simulink model "AUV_MechanicsFullHydrodynamicsVAR"  (R2020b)
settings: Solver=ode23t  StartTime=0.0  StopTime=60  MaxStep=0.01  RelTol=1e-3  EnableMultiTasking=on
PreLoadFcn:
  | AUV_VehicleParameters;
  | Vehicle.Body.markeropacity = 0;
StartFcn:
  | tic;
StopFcn:
  | toc;
model workspace: external: MATLAB File AUV_DataFile_ORIG.m (data not in the file)
undefined symbols (not defined in the file): Environment, Newton, Raphson, smiData, x, X, Y, y, Z
libraries: sm_lib x1595, nesl_utility x51, sharedutil x8, AUVCustomPrimitives_Lib x4, shared6dof x1, aerolibasang x1, aerolibadyn x1
(part 2 of 33)

== system AUV_MechanicsFullHydrodynamicsVAR/AUV/Muiltibody/Cameras ==
  Behind : sm_lib/Frames and Transforms/Reference Frame
  BehindDown : sm_lib/Frames and Transforms/Reference Frame
  BehindUP : sm_lib/Frames and Transforms/Reference Frame
  BehindUPLeft : sm_lib/Frames and Transforms/Reference Frame
  BehindUPRight : sm_lib/Frames and Transforms/Reference Frame
  Side : sm_lib/Frames and Transforms/Reference Frame
  T1 : sm_lib/Frames and Transforms/Rigid Transform  TranslationMethod=Cartesian  TranslationStandardOffset=0  TranslationLengthUnit=m  TranslationStandardAxis=+Z  TranslationCartesianOffset=[-3 0 0]  TranslationROffset=0  TranslationROffsetUnits=m  TranslationZOffset=0  TranslationZOffsetUnits=m  TranslationThetaOffset=0  TranslationThetaOffsetUnits=deg  RotationMethod=None  RotationAngleUnits=deg  RotationStandardAxis=+Z  RotationAngle=0.0  RotationArbitraryAxis=[0 0 1]  FollAlignAxisA=+X  BaseAlignAxisA=+Y  FollAlignAxisB=+Y  BaseAlignAxisB=+Z  RotationSequenceAxes=FollowerAxes  RotationSequence=XYX  RotationSequenceAngles=[0 0 0]  RotationSequenceAnglesUnits=deg  RotationMatrix=[1 0 0; 0 1 0; 0 0 1]
  T2 : sm_lib/Frames and Transforms/Rigid Transform  TranslationMethod=Cartesian  TranslationStandardOffset=0  TranslationLengthUnit=m  TranslationStandardAxis=+Z  TranslationCartesianOffset=[0 0 -3]  TranslationROffset=0  TranslationROffsetUnits=m  TranslationZOffset=0  TranslationZOffsetUnits=m  TranslationThetaOffset=0  TranslationThetaOffsetUnits=deg  RotationMethod=None  RotationAngleUnits=deg  RotationStandardAxis=+Z  RotationAngle=0.0  RotationArbitraryAxis=[0 0 1]  FollAlignAxisA=+X  BaseAlignAxisA=+Y  FollAlignAxisB=+Y  BaseAlignAxisB=+Z  RotationSequenceAxes=FollowerAxes  RotationSequence=XYX  RotationSequenceAngles=[0 0 0]  RotationSequenceAnglesUnits=deg  RotationMatrix=[1 0 0; 0 1 0; 0 0 1]
  T3 : sm_lib/Frames and Transforms/Rigid Transform  TranslationMethod=Cartesian  TranslationStandardOffset=0  TranslationLengthUnit=m  TranslationStandardAxis=+Z  TranslationCartesianOffset=[0 0 -3]  TranslationROffset=0  TranslationROffsetUnits=m  TranslationZOffset=0  TranslationZOffsetUnits=m  TranslationThetaOffset=0  TranslationThetaOffsetUnits=deg  RotationMethod=None  RotationAngleUnits=deg  RotationStandardAxis=+Z  RotationAngle=0.0  RotationArbitraryAxis=[0 0 1]  FollAlignAxisA=+X  BaseAlignAxisA=+Y  FollAlignAxisB=+Y  BaseAlignAxisB=+Z  RotationSequenceAxes=FollowerAxes  RotationSequence=XYX  RotationSequenceAngles=[0 0 0]  RotationSequenceAnglesUnits=deg  RotationMatrix=[1 0 0; 0 1 0; 0 0 1]
  T4 : sm_lib/Frames and Transforms/Rigid Transform  TranslationMethod=Cartesian  TranslationStandardOffset=0  TranslationLengthUnit=m  TranslationStandardAxis=+Z  TranslationCartesianOffset=[0 -2 0]  TranslationROffset=0  TranslationROffsetUnits=m  TranslationZOffset=0  TranslationZOffsetUnits=m  TranslationThetaOffset=0  TranslationThetaOffsetUnits=deg  RotationMethod=None  RotationAngleUnits=deg  RotationStandardAxis=+Z  RotationAngle=0.0  RotationArbitraryAxis=[0 0 1]  FollAlignAxisA=+X  BaseAlignAxisA=+Y  FollAlignAxisB=+Y  BaseAlignAxisB=+Z  RotationSequenceAxes=FollowerAxes  RotationSequence=XYX  RotationSequenceAngles=[0 0 0]  RotationSequenceAnglesUnits=deg  RotationMatrix=[1 0 0; 0 1 0; 0 0 1]
  T5 : sm_lib/Frames and Transforms/Rigid Transform  TranslationMethod=Cartesian  TranslationStandardOffset=0  TranslationLengthUnit=m  TranslationStandardAxis=+Z  TranslationCartesianOffset=[0 -2 0]  TranslationROffset=0  TranslationROffsetUnits=m  TranslationZOffset=0  TranslationZOffsetUnits=m  TranslationThetaOffset=0  TranslationThetaOffsetUnits=deg  RotationMethod=None  RotationAngleUnits=deg  RotationStandardAxis=+Z  RotationAngle=0.0  RotationArbitraryAxis=[0 0 1]  FollAlignAxisA=+X  BaseAlignAxisA=+Y  FollAlignAxisB=+Y  BaseAlignAxisB=+Z  RotationSequenceAxes=FollowerAxes  RotationSequence=XYX  RotationSequenceAngles=[0 0 0]  RotationSequenceAnglesUnits=deg  RotationMatrix=[1 0 0; 0 1 0; 0 0 1]
  T6 : sm_lib/Frames and Transforms/Rigid Transform  TranslationMethod=Cartesian  TranslationStandardOffset=0  TranslationLengthUnit=m  TranslationStandardAxis=+Z  TranslationCartesianOffset=[0 0 -3]  TranslationROffset=0  TranslationROffsetUnits=m  TranslationZOffset=0  TranslationZOffsetUnits=m  TranslationThetaOffset=0  TranslationThetaOffsetUnits=deg  RotationMethod=None  RotationAngleUnits=deg  RotationStandardAxis=+Z  RotationAngle=0.0  RotationArbitraryAxis=[0 0 1]  FollAlignAxisA=+X  BaseAlignAxisA=+Y  FollAlignAxisB=+Y  BaseAlignAxisB=+Z  RotationSequenceAxes=FollowerAxes  RotationSequence=XYX  RotationSequenceAngles=[0 0 0]  RotationSequenceAnglesUnits=deg  RotationMatrix=[1 0 0; 0 1 0; 0 0 1]
  T7 : sm_lib/Frames and Transforms/Rigid Transform  TranslationMethod=Cartesian  TranslationStandardOffset=0  TranslationLengthUnit=m  TranslationStandardAxis=+Z  TranslationCartesianOffset=[0 -3 0]  TranslationROffset=0  TranslationROffsetUnits=m  TranslationZOffset=0  TranslationZOffsetUnits=m  TranslationThetaOffset=0  TranslationThetaOffsetUnits=deg  RotationMethod=None  RotationAngleUnits=deg  RotationStandardAxis=+Z  RotationAngle=0.0  RotationArbitraryAxis=[0 0 1]  FollAlignAxisA=+X  BaseAlignAxisA=+Y  FollAlignAxisB=+Y  BaseAlignAxisB=+Z  RotationSequenceAxes=FollowerAxes  RotationSequence=XYX  RotationSequenceAngles=[0 0 0]  RotationSequenceAnglesUnits=deg  RotationMatrix=[1 0 0; 0 1 0; 0 0 1]
  Top : sm_lib/Frames and Transforms/Reference Frame
  CoM : PMIOPort  Side=Right
  connections:
  T1/LConn1 -- T7/LConn1 -- CoM/RConn1 -- T6/LConn1
  Behind/RConn1 -- T3/RConn1 -- T2/LConn1 -- T1/RConn1
  BehindUP/RConn1 -- T2/RConn1 -- T5/RConn1 -- T4/LConn1
  T3/LConn1 -- BehindDown/RConn1
  BehindUPLeft/RConn1 -- T4/RConn1
  T5/LConn1 -- BehindUPRight/RConn1
  Top/RConn1 -- T6/RConn1
  Side/RConn1 -- T7/RConn1

== system AUV_MechanicsFullHydrodynamicsVAR/AUV/Muiltibody/Hydro Forces & Moments ==
  Bus Element In : Inport  PortName=HydroForces  Element=Buoyancy.BForceZ
  Bus Element In1 : Inport  PortName=HydroForces  Element=LiftNDrag.LDForcesXYZ
  Bus Element In2 : Inport  PortName=HydroForces  Element=LiftNDrag.LDMomentsXYZ
  Bus Element In3 : Inport  PortName=HydroForces  Element=AddedMass.AMForcesXYZ
  Bus Element In4 : Inport  PortName=HydroForces  Element=AddedMass.AMMomentsXYZ
  Bus Element In5 : Inport  PortName=HydroForces  Element=AddedMass.CMomentsXYZ
  Bus Element In6 : Inport  PortName=HydroForces  Element=AddedMass.CForcesXYZ
  Added Mass Coriolis : Subsystem
  Added Mass Forces : Subsystem
  Buoyancy Force : Subsystem
  Lift and Drag Forces : Subsystem
  CoM : PMIOPort  Side=Right
  CoB : PMIOPort  Port=2  Side=Right
  wires:
  Bus Element In/1 -> Buoyancy Force/1(B)
  Bus Element In1/1 -> Lift and Drag Forces/1(Fxyz)
  Bus Element In2/1 -> Lift and Drag Forces/2(Mxyz)
  Bus Element In3/1 -> Added Mass Forces/1(Fxyz)
  Bus Element In4/1 -> Added Mass Forces/2(Mxyz)
  Bus Element In5/1 -> Added Mass Coriolis/2(Mxyz)
  Bus Element In6/1 -> Added Mass Coriolis/1(Fxyz)
  connections:
  CoB/RConn1 -- Buoyancy Force/RConn1
  Lift and Drag Forces/RConn1 -- Added Mass Coriolis/RConn1 -- Added Mass Forces/RConn1 -- CoM/RConn1

== system AUV_MechanicsFullHydrodynamicsVAR/AUV/Muiltibody/World ==
  Mechanism Configuration : sm_lib/Utilities/Mechanism Configuration  UniformGravity=Constant  GravityVector=[0 0 Environment.gravity]  GravityUnits=m/s^2  LinearizationDelta=0.001
  Sea Floor : Subsystem
  Solver Configuration : nesl_utility/Solver Configuration  PhysicalDomain=network_engine_domain  SubClassName=solver  LeftPortType=input  RightPortType=generic  Tones=[]  Harmonics=[]  SimulateNoise=off  Profile=off  UseLocalSampling=off  EnableSwitchedLinearOptims=on  FrequencyDomain=off  UseCCode=off  RelTol=0.001  AbsTol=1e-06  MinStep=1e-09  ToWorkspace=off  RevertToSquareIcSolve=off  NumHomotopyIterations=100  PhasorMode=off  PhasorModeNumHarmonics=1  DoDC=off  ResidualTolerance=1e-09  UseLocalSolver=off  LocalSolverChoice=NE_BACKWARD_EULER_ADVANCER  LocalSolverSampleTime=0.001  DoFixedCost=off  MaxNonlinIter=3  MaxModeIter=2  LinearAlgebra=Sparse  EquationFormulation=NE_TIME_EF  DelaysMemoryBudget=1024  AutomaticFiltering=on  FilteringTimeConstant=0.001  PartitionStorageMethod=AS_NEEDED  PartitionMemoryBudget=1024  PartitionMethod=FAST
  World Frame --> e NED : sm_lib/Frames and Transforms/World Frame
  W : PMIOPort  Side=Right
  connections:
  World Frame --> e NED/RConn1 -- W/RConn1 -- Sea Floor/LConn1 -- Mechanism Configuration/RConn1 -- Solver Configuration/RConn1

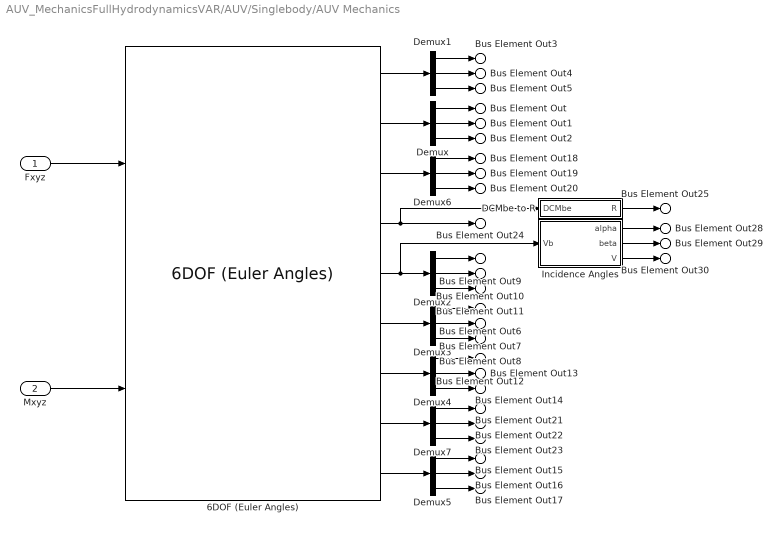
== system AUV_MechanicsFullHydrodynamicsVAR/AUV/Singlebody/AUV Mechanics ==
  Fxyz : Inport
  Mxyz : Inport  Port=2
  6DOF (Euler Angles) : shared6dof/6DOF (Euler Angles)  units=Metric (MKS)  mtype=Fixed  rep=Euler Angles  xme_0=Vehicle.InitCond.position  Vm_0=Vehicle.InitCond.velocity  eul_0=Vehicle.InitCond.EulerXYZrad  pm_0=Vehicle.InitCond.rotrates  mass_0=Vehicle.Body.Full.mass  mass_e=0.5  mass_f=2.0  inertia=Vehicle.Body.Full.Inertia  inertia_e=eye(3)  inertia_f=2*eye(3)  k_quat=1.0  vre_flag=on  abi_flag=on  aMode=0  xme_statename=''  Vm_statename=''  eul_statename=''  quat_statename=''  pm_statename=''  mass_statename=''
      settings: SourceProductBaseCode=AE,PW,MT,UV,VE,VP
  DCMbe to R : Subsystem
  Demux{,1..7} (8 alike) : Demux  Outputs=3
  Incidence Angles : Subsystem
  Bus Element Out : Outport  PortName=CoM  Element=World.Xe.X
  Bus Element Out1 : Outport  PortName=CoM  Element=World.Xe.Y
  Bus Element Out2 : Outport  PortName=CoM  Element=World.Xe.Z
  Bus Element Out3 : Outport  PortName=CoM  Element=World.Ve.Vx
  Bus Element Out4 : Outport  PortName=CoM  Element=World.Ve.Vy
  Bus Element Out5 : Outport  PortName=CoM  Element=World.Ve.Vz
  Bus Element Out25 : Outport  PortName=CoM  Element=World.R
  Bus Element Out6 : Outport  PortName=CoM  Element=Body.wb.p
  Bus Element Out7 : Outport  PortName=CoM  Element=Body.wb.q
  Bus Element Out8 : Outport  PortName=CoM  Element=Body.wb.r
  Bus Element Out9 : Outport  PortName=CoM  Element=Body.Vb.u
  Bus Element Out10 : Outport  PortName=CoM  Element=Body.Vb.v
  Bus Element Out11 : Outport  PortName=CoM  Element=Body.Vb.w
  Bus Element Out12 : Outport  PortName=CoM  Element=Body.dwbdt.pdot
  Bus Element Out13 : Outport  PortName=CoM  Element=Body.dwbdt.qdot
  Bus Element Out14 : Outport  PortName=CoM  Element=Body.dwbdt.rdot
  Bus Element Out15 : Outport  PortName=CoM  Element=Body.Abe.ax
  Bus Element Out16 : Outport  PortName=CoM  Element=Body.Abe.ay
  Bus Element Out17 : Outport  PortName=CoM  Element=Body.Abe.az
  Bus Element Out18 : Outport  PortName=CoM  Element=Derived.Euler.phi
  Bus Element Out19 : Outport  PortName=CoM  Element=Derived.Euler.theta
  Bus Element Out20 : Outport  PortName=CoM  Element=Derived.Euler.psi
  Bus Element Out21 : Outport  PortName=CoM  Element=Derived.Body.Abb.Abbx
  Bus Element Out22 : Outport  PortName=CoM  Element=Derived.Body.Abb.Abby
  Bus Element Out23 : Outport  PortName=CoM  Element=Derived.Body.Abb.Abbz
  Bus Element Out28 : Outport  PortName=CoM  Element=Derived.Body.Incidences.alpha
  Bus Element Out29 : Outport  PortName=CoM  Element=Derived.Body.Incidences.beta
  Bus Element Out30 : Outport  PortName=CoM  Element=Derived.Body.V
  Bus Element Out24 : Outport  PortName=CoM  Element=Derived.World.DCMbe
  wires:
  Fxyz/1 -> 6DOF (Euler Angles)/1
  6DOF (Euler Angles)/2 -> Demux/1
  Mxyz/1 -> 6DOF (Euler Angles)/2
  Demux/2 -> Bus Element Out1/1
  Demux/1 -> Bus Element Out/1
  Demux/3 -> Bus Element Out2/1
  6DOF (Euler Angles)/1 -> Demux1/1
  Demux1/1 -> Bus Element Out3/1
  Demux1/2 -> Bus Element Out4/1
  Demux1/3 -> Bus Element Out5/1
  6DOF (Euler Angles)/5 -> Demux2/1, Incidence Angles/1(Vb)
  6DOF (Euler Angles)/6 -> Demux3/1
  Demux3/1 -> Bus Element Out6/1
  Demux3/2 -> Bus Element Out7/1
  Demux3/3 -> Bus Element Out8/1
  Demux2/1 -> Bus Element Out9/1
  Demux2/2 -> Bus Element Out10/1
  Demux2/3 -> Bus Element Out11/1
  6DOF (Euler Angles)/7 -> Demux4/1
  Demux4/1 -> Bus Element Out12/1
  Demux4/2 -> Bus Element Out13/1
  Demux4/3 -> Bus Element Out14/1
  6DOF (Euler Angles)/9 -> Demux5/1
  Demux5/1 -> Bus Element Out15/1
  Demux5/2 -> Bus Element Out16/1
  Demux5/3 -> Bus Element Out17/1
  6DOF (Euler Angles)/3 -> Demux6/1
  Demux6/1 -> Bus Element Out18/1
  Demux6/2 -> Bus Element Out19/1
  Demux6/3 -> Bus Element Out20/1
  6DOF (Euler Angles)/8 -> Demux7/1
  Demux7/1 -> Bus Element Out21/1
  Demux7/2 -> Bus Element Out22/1
  Demux7/3 -> Bus Element Out23/1
  6DOF (Euler Angles)/4 -> Bus Element Out24/1, DCMbe to R/1(DCMbe)
  Incidence Angles/1(alpha) -> Bus Element Out28/1
  Incidence Angles/2(beta) -> Bus Element Out29/1
  Incidence Angles/3(V) -> Bus Element Out30/1
  DCMbe to R/1(R) -> Bus Element Out25/1

== system AUV_MechanicsFullHydrodynamicsVAR/AUV/Singlebody/Hydro Forces & Moments ==
  Bus Element In : Inport  PortName=HydroForces  Element=Buoyancy.BForceZ
  Bus Element In1 : Inport  PortName=HydroForces  Element=Weight.WForceZ
  Bus Element In3 : Inport  PortName=HydroForces  Element=AddedMass.AMForcesXYZ
  Bus Element In4 : Inport  PortName=HydroForces  Element=AddedMass.AMMomentsXYZ
  Bus Element In5 : Inport  PortName=HydroForces  Element=AddedMass.CForcesXYZ
  Bus Element In6 : Inport  PortName=HydroForces  Element=AddedMass.CMomentsXYZ
  Bus Element In7 : Inport  PortName=HydroForces  Element=LiftNDrag.LDForcesXYZ
  Bus Element In8 : Inport  PortName=HydroForces  Element=LiftNDrag.LDMomentsXYZ
  Bus Element In2 : Inport  Port=2  PortName=CoM  Element=Derived.World.DCMbe
  Added Mass Forces : Subsystem
  Hydrostatic Forces : Subsystem
  Lift and Drag Forces : Subsystem
  Sum : Sum  Inputs=+++
  Sum1 : Sum  Inputs=+++
  Fxyz : Outport
  Mxyz : Outport  Port=2
  wires:
  Bus Element In2/1 -> Hydrostatic Forces/1(DCM)
  Bus Element In/1 -> Hydrostatic Forces/2(Bz)
  Bus Element In1/1 -> Hydrostatic Forces/3(Wz)
  Bus Element In3/1 -> Added Mass Forces/1(AMFxyz)
  Bus Element In4/1 -> Added Mass Forces/2(AMMxyz)
  Bus Element In5/1 -> Added Mass Forces/3(AMCFxyz)
  Bus Element In6/1 -> Added Mass Forces/4(AMCMxyz)
  Bus Element In7/1 -> Lift and Drag Forces/1(LDFxyz)
  Bus Element In8/1 -> Lift and Drag Forces/2(LDMxyz)
  Lift and Drag Forces/1(Fxyz) -> Sum/2
  Sum/1 -> Fxyz/1
  Hydrostatic Forces/1(Fxyz) -> Sum/1
  Added Mass Forces/1(Fxyz) -> Sum/3
  Sum1/1 -> Mxyz/1
  Lift and Drag Forces/2(Mxyz) -> Sum1/2
  Hydrostatic Forces/2(Mxyz) -> Sum1/1
  Added Mass Forces/2(Mxyz) -> Sum1/3

== system AUV_MechanicsFullHydrodynamicsVAR/AUV/Singlebody/Propellers & Thrusters ==
  Bus Element In : Inport  PortName=Actuators  Element=Propellers.PPf
  Bus Element In1 : Inport  PortName=Actuators  Element=Propellers.SPf
  Bus Element In2 : Inport  PortName=Actuators  Element=Thrusters.BHTf
  Bus Element In3 : Inport  PortName=Actuators  Element=Thrusters.BVTf
  Bus Element In4 : Inport  PortName=Actuators  Element=Thrusters.SHTf
  Bus Element In5 : Inport  PortName=Actuators  Element=Thrusters.SVTf
  Horizontal Tunnel Thrusters : Subsystem
  Main Propellers : Subsystem
  Sum : Sum  Inputs=+++
  Sum1 : Sum  Inputs=+++
  Vertical Tunnel Thrusters : Subsystem
  Fxyz : Outport
  Mxyz : Outport  Port=2
  wires:
  Bus Element In1/1 -> Main Propellers/1(SPf)
  Bus Element In/1 -> Main Propellers/2(PPf)
  Bus Element In3/1 -> Vertical Tunnel Thrusters/1(BVTf)
  Bus Element In5/1 -> Vertical Tunnel Thrusters/2(SVTf)
  Bus Element In2/1 -> Horizontal Tunnel Thrusters/1(BHTf)
  Bus Element In4/1 -> Horizontal Tunnel Thrusters/2(SHTf)
  Horizontal Tunnel Thrusters/1(Fxyz) -> Sum/2
  Sum/1 -> Fxyz/1
  Main Propellers/1(Fxyz) -> Sum/1
  Vertical Tunnel Thrusters/1(Fxyz) -> Sum/3
  Sum1/1 -> Mxyz/1
  Horizontal Tunnel Thrusters/2(Mxyz) -> Sum1/2
  Main Propellers/2(Mxyz) -> Sum1/1
  Vertical Tunnel Thrusters/2(Mxyz) -> Sum1/3

== system AUV_MechanicsFullHydrodynamicsVAR/Hydrostatic & Hydrodynamic Effects/Added Mass Forces/Added Mass ==
  note: NOTE:
      | The forces due to added mass will me applied as external
      | forces, so they will oppose the direction of the accelerations
      |
      | $M_{rb}\dot{\nu}+C_{rb}(\nu)\nu= F_{propulsion} - M_a\dot{\nu}-C_a(\nu)\nu-D(\nu)\nu$
  Ma : Inport
  Abb : Inport  Port=2
  dwbdt : Inport  Port=3
  Demux : Demux  Outputs=[3,3]
  Gain : Gain  Gain=-1
  LPfilter : Subsystem
  Ma*[Abb,dwbdt]' : Product  Multiplication=Matrix(*)
  "[Abb,dwbdt]'" : Concatenate  Mode=Multidimensional array
  Fxyz : Outport
  Mxyz : Outport  Port=2
  wires:
  dwbdt/1 -> "[Abb,dwbdt]'"/2
  "[Abb,dwbdt]'"/1 -> Ma*[Abb,dwbdt]'/2
  Demux/2 -> Mxyz/1
  Ma/1 -> Ma*[Abb,dwbdt]'/1
  Abb/1 -> "[Abb,dwbdt]'"/1
  Demux/1 -> Fxyz/1
  Ma*[Abb,dwbdt]'/1 -> LPfilter/1(in)
  LPfilter/1(out) -> Gain/1
  Gain/1 -> Demux/1

== system AUV_MechanicsFullHydrodynamicsVAR/Hydrostatic & Hydrodynamic Effects/Added Mass Forces/Coriolis ==
  note: Coriolis matrix
  note: NOTE:
      | It is important to mention that the coriolis matrix due to added mass
      | computed here includes the de-stabilizing Munk-moment .
      | This moment acts to turn the vehicle perpendicular to the flow, and it
      | is most dominant for slender body vehicles in pitch and yaw when the
      | lateral velocities are non-zero.
      | This de-stabilizing effect will need to be accounted for in the design
      | of the control algorithm.
  Vb : Inport
  wb : Inport  Port=2
  Ma : Inport  Port=3
  Ca(V) : Subsystem
  Ca(V)*[Vb,wb]' : Product  Multiplication=Matrix(*)
  Demux : Demux  Outputs=6
  Demux1 : Demux  Outputs=[3,3]
  Gain : Gain  Gain=-1
  Ma*[Vb,wb]' : Product  Multiplication=Matrix(*)
  "[Vb,wb]'" : Concatenate  Mode=Multidimensional array
  Fxyz : Outport
  Mxyz : Outport  Port=2
  wires:
  Ma/1 -> Ma*[Vb,wb]'/1
  Vb/1 -> "[Vb,wb]'"/1
  wb/1 -> "[Vb,wb]'"/2
  "[Vb,wb]'"/1 -> Ca(V)*[Vb,wb]'/2, Ma*[Vb,wb]'/2
  Ma*[Vb,wb]'/1 -> Demux/1
  Demux/1 -> Ca(V)/1(a1)  "a1"
  Demux/2 -> Ca(V)/2(a2)  "a2"
  Demux/3 -> Ca(V)/3(a3)  "a3"
  Demux/4 -> Ca(V)/4(b1)  "b1"
  Demux/5 -> Ca(V)/5(b2)  "b2"
  Demux/6 -> Ca(V)/6(b3)  "b3"
  Ca(V)/1(Ca(V)) -> Ca(V)*[Vb,wb]'/1
  Ca(V)*[Vb,wb]'/1 -> Gain/1
  Demux1/1 -> Fxyz/1
  Demux1/2 -> Mxyz/1
  Gain/1 -> Demux1/1

== system AUV_MechanicsFullHydrodynamicsVAR/Hydrostatic & Hydrodynamic Effects/Lift and Drag Forces/Hydrodynamic Coefficients ==
  alpha,beta : Inport
  wb : Inport  Port=2
  Vb : Inport  Port=3
  Body Rate Damping : Subsystem
  Demux : Demux  Outputs=2
  Drag and Lift Coefficients : Subsystem
  Sum : Sum  Inputs=++|
  rad to deg : UnitConversion
  Coeff : Outport
  wires:
  alpha,beta/1 -> rad to deg/1
  rad to deg/1 -> Demux/1
  Demux/1 -> Body Rate Damping/3(alpha), Drag and Lift Coefficients/1(alpha)
  Demux/2 -> Drag and Lift Coefficients/2(beta)
  Vb/1 -> Body Rate Damping/1(Vb)
  wb/1 -> Body Rate Damping/2(pqr)
  Drag and Lift Coefficients/1(coeff) -> Sum/2
  Body Rate Damping/1(coeff) -> Sum/1
  Sum/1 -> Coeff/1

== system AUV_MechanicsFullHydrodynamicsVAR/AUV/Muiltibody/AUV Mechanics/AUVBody ==
  BowHorThrusterTunnel : Subsystem
      settings: PortSchema="{\"entries\":[{\"content\":{\"sides\":[{\"content\":{\"connectorIds\":[]},\"type\":\"ConnectorPlacement.EquallySpacedRectSide\",\"uuid\":\"4ed08382-faad-44b6-b48b-55aec1852bc8\"},{\"content\":{\"connectorIds\":[\"RConn1\"],\"side\":\"RIGHT\"},\"type\":\"ConnectorPlacement.EquallySpacedRectSide\",\"uuid\":\"f82da02f-1c57-4ab6-ab88-6cf954e3e010\"},{\"content\":{\"connectorIds\":[\"LConn1\"],\"side\":\"TOP\"},\"type\":\"ConnectorPlacement.EquallySpacedRectSide\",\"uuid\":\"303110cd-3491-4a84-90e7-28fdba545389\"}]},\"type\":\"ConnectorPlacement.EquallySpacedConnector\",\"uuid\":\"9acf980f-250a-4e2c-8e72-208e68ccad03\"}],\"packageUris\":[\"http://schema.mathworks.com/mf0/Connector/19700101\"],\"version\":\"1.0\"}"
      mask Display: image('HorizontalTunnelNSensors.png')
  BowHullCap : Subsystem
      settings: PortSchema="{\"entries\":[{\"content\":{\"sides\":[{\"content\":{\"connectorIds\":[\"LConn1\"]},\"type\":\"ConnectorPlacement.EquallySpacedRectSide\",\"uuid\":\"ee174d83-7ec9-4f78-977a-5ac618f84910\"},{\"content\":{\"connectorIds\":[],\"side\":\"RIGHT\"},\"type\":\"ConnectorPlacement.EquallySpacedRectSide\",\"uuid\":\"b1f8772f-a994-4bc2-984b-3dde78400d8f\"},{\"content\":{\"connectorIds\":[\"LConn2\"],\"side\":\"TOP\"},\"type\":\"ConnectorPlacement.EquallySpacedRectSide\",\"uuid\":\"f9256764-d20c-453c-9456-9dc5ed28a8dc\"}]},\"type\":\"ConnectorPlacement.EquallySpacedConnector\",\"uuid\":\"1072f53a-ce7b-4a5a-9466-cf066be5f153\"}],\"packageUris\":[\"http://schema.mathworks.com/mf0/Connector/19700101\"],\"version\":\"1.0\"}"
      mask Display: image('BowHullCapNSensors.png')
  BowVerThrusterTunnel : Subsystem
      settings: PortSchema="{\"entries\":[{\"content\":{\"sides\":[{\"content\":{\"connectorIds\":[]},\"type\":\"ConnectorPlacement.EquallySpacedRectSide\",\"uuid\":\"1a213aad-fe79-4629-9576-af927b73c724\"},{\"content\":{\"connectorIds\":[\"RConn1\"],\"side\":\"RIGHT\"},\"type\":\"ConnectorPlacement.EquallySpacedRectSide\",\"uuid\":\"bc8c7819-b1a4-4404-9606-1fc6a621b846\"},{\"content\":{\"connectorIds\":[\"LConn1\"],\"side\":\"TOP\"},\"type\":\"ConnectorPlacement.EquallySpacedRectSide\",\"uuid\":\"4fef86ac-72f6-48ad-8cd5-107d8fb60770\"}]},\"type\":\"ConnectorPlacement.EquallySpacedConnector\",\"uuid\":\"055cc73a-4714-4bde-94dc-e41324e94198\"}],\"packageUris\":[\"http://schema.mathworks.com/mf0/Connector/19700101\"],\"version\":\"1.0\"}"
      mask Display: image('VerticalTunnel.png')
  MainHull : Subsystem
      settings: PortSchema="{\"entries\":[{\"content\":{\"sides\":[{\"content\":{\"connectorIds\":[\"LConn1\",\"LConn2\"]},\"type\":\"ConnectorPlacement.EquallySpacedRectSide\",\"uuid\":\"76cfb896-16da-4ec2-9221-4dfc6f13d712\"},{\"content\":{\"connectorIds\":[\"RConn1\"],\"side\":\"RIGHT\"},\"type\":\"ConnectorPlacement.EquallySpacedRectSide\",\"uuid\":\"9107ed06-22d1-41c2-9864-d0faf2c3be22\"},{\"content\":{\"connectorIds\":[\"LConn3\"],\"side\":\"TOP\"},\"type\":\"ConnectorPlacement.EquallySpacedRectSide\",\"uuid\":\"11b30dc3-5e1b-4eeb-82e1-3f429735ec8f\"}]},\"type\":\"ConnectorPlacement.EquallySpacedConnector\",\"uuid\":\"22417ec0-808b-431c-ad0b-85484074bdac\"}],\"packageUris\":[\"http://schema.mathworks.com/mf0/Connector/19700101\"],\"version\":\"1.0\"}"
      mask Display: image('HullNSensors.png',[0,0.05,1,0.9])
  ReferenceFrame : sm_lib/Frames and Transforms/Reference Frame
  SternHorThrusterTunnel : Subsystem
      settings: PortSchema="{\"entries\":[{\"content\":{\"sides\":[{\"content\":{\"connectorIds\":[]},\"type\":\"ConnectorPlacement.EquallySpacedRectSide\",\"uuid\":\"1a213aad-fe79-4629-9576-af927b73c724\"},{\"content\":{\"connectorIds\":[\"RConn1\"],\"side\":\"RIGHT\"},\"type\":\"ConnectorPlacement.EquallySpacedRectSide\",\"uuid\":\"bc8c7819-b1a4-4404-9606-1fc6a621b846\"},{\"content\":{\"connectorIds\":[\"LConn1\"],\"side\":\"TOP\"},\"type\":\"ConnectorPlacement.EquallySpacedRectSide\",\"uuid\":\"4fef86ac-72f6-48ad-8cd5-107d8fb60770\"}]},\"type\":\"ConnectorPlacement.EquallySpacedConnector\",\"uuid\":\"055cc73a-4714-4bde-94dc-e41324e94198\"}],\"packageUris\":[\"http://schema.mathworks.com/mf0/Connector/19700101\"],\"version\":\"1.0\"}"
      mask Display: image('HorizontalTunnel.png')
  SternHullCap : Subsystem
      settings: PortSchema="{\"entries\":[{\"content\":{\"sides\":[{\"content\":{\"connectorIds\":[]},\"type\":\"ConnectorPlacement.EquallySpacedRectSide\",\"uuid\":\"4ed08382-faad-44b6-b48b-55aec1852bc8\"},{\"content\":{\"connectorIds\":[],\"side\":\"RIGHT\"},\"type\":\"ConnectorPlacement.EquallySpacedRectSide\",\"uuid\":\"f82da02f-1c57-4ab6-ab88-6cf954e3e010\"},{\"content\":{\"connectorIds\":[\"LConn1\"],\"side\":\"TOP\"},\"type\":\"ConnectorPlacement.EquallySpacedRectSide\",\"uuid\":\"303110cd-3491-4a84-90e7-28fdba545389\"}]},\"type\":\"ConnectorPlacement.EquallySpacedConnector\",\"uuid\":\"9acf980f-250a-4e2c-8e72-208e68ccad03\"}],\"packageUris\":[\"http://schema.mathworks.com/mf0/Connector/19700101\"],\"version\":\"1.0\"}"
      mask Display: image('SternHullCapNSensor.png')
  SternVerThrusterTunnel : Subsystem
      settings: PortSchema="{\"entries\":[{\"content\":{\"sides\":[{\"content\":{\"connectorIds\":[]},\"type\":\"ConnectorPlacement.EquallySpacedRectSide\",\"uuid\":\"1a213aad-fe79-4629-9576-af927b73c724\"},{\"content\":{\"connectorIds\":[\"RConn1\"],\"side\":\"RIGHT\"},\"type\":\"ConnectorPlacement.EquallySpacedRectSide\",\"uuid\":\"bc8c7819-b1a4-4404-9606-1fc6a621b846\"},{\"content\":{\"connectorIds\":[\"LConn1\"],\"side\":\"TOP\"},\"type\":\"ConnectorPlacement.EquallySpacedRectSide\",\"uuid\":\"4fef86ac-72f6-48ad-8cd5-107d8fb60770\"}]},\"type\":\"ConnectorPlacement.EquallySpacedConnector\",\"uuid\":\"055cc73a-4714-4bde-94dc-e41324e94198\"}],\"packageUris\":[\"http://schema.mathworks.com/mf0/Connector/19700101\"],\"version\":\"1.0\"}"
      mask Display: image('VerticalTunnel.png')
  BHT : PMIOPort  Side=Left
  BVT : PMIOPort  Port=2  Side=Right
  W : PMIOPort  Port=3  Side=Left
  IMU : PMIOPort  Port=4  Side=Right
  SP : PMIOPort  Port=5  Side=Right
  PP : PMIOPort  Port=6  Side=Left
  SVT : PMIOPort  Port=7  Side=Right
  SHT : PMIOPort  Port=8  Side=Left
  connections:
  BowHullCap/LConn2 -- SternHullCap/LConn1 -- SternHorThrusterTunnel/LConn1 -- SternVerThrusterTunnel/LConn1 -- MainHull/LConn3 -- ReferenceFrame/RConn1 -- BowVerThrusterTunnel/LConn1 -- BowHorThrusterTunnel/LConn1
  W/RConn1 -- BowHullCap/LConn1
  BHT/RConn1 -- BowHorThrusterTunnel/RConn1
  BVT/RConn1 -- BowVerThrusterTunnel/RConn1
  SternVerThrusterTunnel/RConn1 -- SVT/RConn1
  SHT/RConn1 -- SternHorThrusterTunnel/RConn1
  MainHull/LConn1 -- IMU/RConn1
  SP/RConn1 -- MainHull/LConn2
  PP/RConn1 -- MainHull/RConn1

== system AUV_MechanicsFullHydrodynamicsVAR/AUV/Muiltibody/AUV Mechanics/AlignFrames ==
  Align Vehicle with NED : sm_lib/Frames and Transforms/Rigid Transform  TranslationMethod=None  TranslationStandardOffset=0  TranslationLengthUnit=m  TranslationStandardAxis=+Z  TranslationCartesianOffset=[0 0 0]  TranslationROffset=0  TranslationROffsetUnits=m  TranslationZOffset=0  TranslationZOffsetUnits=m  TranslationThetaOffset=0  TranslationThetaOffsetUnits=deg  RotationMethod=RotationSequence  RotationAngleUnits=deg  RotationStandardAxis=+Z  RotationAngle=0.0  RotationArbitraryAxis=[0 0 1]  FollAlignAxisA=+X  BaseAlignAxisA=+Y  FollAlignAxisB=+Y  BaseAlignAxisB=+Z  RotationSequenceAxes=BaseAxes  RotationSequence=YXZ  RotationSequenceAngles=[90 -90 0]  RotationSequenceAnglesUnits=deg  RotationMatrix=[1 0 0; 0 1 0; 0 0 1]
  CoB Location Marker : sm_lib/Body Elements/Graphic  GraphicType=Marker  MarkerShape=Frame  MarkerSize=20  GraphicVisPropType=SimpleVisualProperties  GraphicDiffuseColor=[0.0 0.9529412 0.0]  GraphicSpecularColor=[0.5 0.5 0.5 1.0]  GraphicAmbientColor=[0.15 0.15 0.15 1.0]  GraphicEmissiveColor=[0.0 0.0 0.0 1.0]  GraphicShininess=75  GraphicOpacity=Vehicle.Body.markeropacity
  CoM Location Marker : sm_lib/Body Elements/Graphic  GraphicType=Marker  MarkerShape=Frame  MarkerSize=20  GraphicVisPropType=SimpleVisualProperties  GraphicDiffuseColor=[0.85882354 0.0 0.0]  GraphicSpecularColor=[0.5 0.5 0.5 1.0]  GraphicAmbientColor=[0.15 0.15 0.15 1.0]  GraphicEmissiveColor=[0.0 0.0 0.0 1.0]  GraphicShininess=75  GraphicOpacity=Vehicle.Body.markeropacity
  Translate to Vehicle CoB : sm_lib/Frames and Transforms/Rigid Transform  TranslationMethod=Cartesian  TranslationStandardOffset=0  TranslationLengthUnit=m  TranslationStandardAxis=+Z  TranslationCartesianOffset=Vehicle.Body.Full.CoB  TranslationROffset=0  TranslationROffsetUnits=m  TranslationZOffset=0  TranslationZOffsetUnits=m  TranslationThetaOffset=0  TranslationThetaOffsetUnits=deg  RotationMethod=None  RotationAngleUnits=deg  RotationStandardAxis=+Z  RotationAngle=0.0  RotationArbitraryAxis=[0 0 1]  FollAlignAxisA=+X  BaseAlignAxisA=+Y  FollAlignAxisB=+Y  BaseAlignAxisB=+Z  RotationSequenceAxes=FollowerAxes  RotationSequence=XYX  RotationSequenceAngles=[0 0 0]  RotationSequenceAnglesUnits=deg  RotationMatrix=[1 0 0; 0 1 0; 0 0 1]
  Translate to Vehicle CoM : sm_lib/Frames and Transforms/Rigid Transform  TranslationMethod=Cartesian  TranslationStandardOffset=0  TranslationLengthUnit=m  TranslationStandardAxis=+Z  TranslationCartesianOffset=Vehicle.Body.Full.CoM  TranslationROffset=0  TranslationROffsetUnits=m  TranslationZOffset=0  TranslationZOffsetUnits=m  TranslationThetaOffset=0  TranslationThetaOffsetUnits=deg  RotationMethod=None  RotationAngleUnits=deg  RotationStandardAxis=+Z  RotationAngle=0.0  RotationArbitraryAxis=[0 0 1]  FollAlignAxisA=+X  BaseAlignAxisA=+Y  FollAlignAxisB=+Y  BaseAlignAxisB=+Z  RotationSequenceAxes=FollowerAxes  RotationSequence=XYX  RotationSequenceAngles=[0 0 0]  RotationSequenceAnglesUnits=deg  RotationMatrix=[1 0 0; 0 1 0; 0 0 1]
  CoM : PMIOPort  Side=Left
  CoB : PMIOPort  Port=2  Side=Left
  W : PMIOPort  Port=3  Side=Right
  connections:
  Translate to Vehicle CoM/LConn1 -- Translate to Vehicle CoB/LConn1 -- Align Vehicle with NED/LConn1
  CoB Location Marker/RConn1 -- Translate to Vehicle CoB/RConn1 -- CoB/RConn1
  W/RConn1 -- Align Vehicle with NED/RConn1
  CoM Location Marker/RConn1 -- CoM/RConn1 -- Translate to Vehicle CoM/RConn1

== system AUV_MechanicsFullHydrodynamicsVAR/AUV/Muiltibody/AUV Mechanics/BowHorThruster ==
  ReferenceFrame : sm_lib/Frames and Transforms/Reference Frame
  T1 : sm_lib/Frames and Transforms/Rigid Transform  TranslationMethod=Cartesian  TranslationStandardOffset=0  TranslationLengthUnit=m  TranslationStandardAxis=+Z  TranslationCartesianOffset=smiData.RigidTransform(10).translation  TranslationROffset=0  TranslationROffsetUnits=m  TranslationZOffset=0  TranslationZOffsetUnits=m  TranslationThetaOffset=0  TranslationThetaOffsetUnits=deg  RotationMethod=ArbitraryAxis  RotationAngleUnits=rad  RotationStandardAxis=+Z  RotationAngle=smiData.RigidTransform(10).angle  RotationArbitraryAxis=smiData.RigidTransform(10).axis  FollAlignAxisA=+X  BaseAlignAxisA=+Y  FollAlignAxisB=+Y  BaseAlignAxisB=+Z  RotationSequenceAxes=FollowerAxes  RotationSequence=XYX  RotationSequenceAngles=[0 0 0]  RotationSequenceAnglesUnits=deg  RotationMatrix=[1 0 0; 0 1 0; 0 0 1]
  T2 : sm_lib/Frames and Transforms/Rigid Transform  TranslationMethod=Cartesian  TranslationStandardOffset=0  TranslationLengthUnit=m  TranslationStandardAxis=+Z  TranslationCartesianOffset=smiData.RigidTransform(108).translation  TranslationROffset=0  TranslationROffsetUnits=m  TranslationZOffset=0  TranslationZOffsetUnits=m  TranslationThetaOffset=0  TranslationThetaOffsetUnits=deg  RotationMethod=ArbitraryAxis  RotationAngleUnits=rad  RotationStandardAxis=+Z  RotationAngle=smiData.RigidTransform(108).angle  RotationArbitraryAxis=smiData.RigidTransform(108).axis  FollAlignAxisA=+X  BaseAlignAxisA=+Y  FollAlignAxisB=+Y  BaseAlignAxisB=+Z  RotationSequenceAxes=FollowerAxes  RotationSequence=XYX  RotationSequenceAngles=[0 0 0]  RotationSequenceAnglesUnits=deg  RotationMatrix=[1 0 0; 0 1 0; 0 0 1]
  T3 : sm_lib/Frames and Transforms/Rigid Transform  TranslationMethod=Cartesian  TranslationStandardOffset=0  TranslationLengthUnit=m  TranslationStandardAxis=+Z  TranslationCartesianOffset=smiData.RigidTransform(109).translation  TranslationROffset=0  TranslationROffsetUnits=m  TranslationZOffset=0  TranslationZOffsetUnits=m  TranslationThetaOffset=0  TranslationThetaOffsetUnits=deg  RotationMethod=ArbitraryAxis  RotationAngleUnits=rad  RotationStandardAxis=+Z  RotationAngle=smiData.RigidTransform(109).angle  RotationArbitraryAxis=smiData.RigidTransform(109).axis  FollAlignAxisA=+X  BaseAlignAxisA=+Y  FollAlignAxisB=+Y  BaseAlignAxisB=+Z  RotationSequenceAxes=FollowerAxes  RotationSequence=XYX  RotationSequenceAngles=[0 0 0]  RotationSequenceAnglesUnits=deg  RotationMatrix=[1 0 0; 0 1 0; 0 0 1]
  T4 : sm_lib/Frames and Transforms/Rigid Transform  TranslationMethod=Cartesian  TranslationStandardOffset=0  TranslationLengthUnit=m  TranslationStandardAxis=+Z  TranslationCartesianOffset=smiData.RigidTransform(110).translation  TranslationROffset=0  TranslationROffsetUnits=m  TranslationZOffset=0  TranslationZOffsetUnits=m  TranslationThetaOffset=0  TranslationThetaOffsetUnits=deg  RotationMethod=ArbitraryAxis  RotationAngleUnits=rad  RotationStandardAxis=+Z  RotationAngle=smiData.RigidTransform(110).angle  RotationArbitraryAxis=smiData.RigidTransform(110).axis  FollAlignAxisA=+X  BaseAlignAxisA=+Y  FollAlignAxisB=+Y  BaseAlignAxisB=+Z  RotationSequenceAxes=FollowerAxes  RotationSequence=XYX  RotationSequenceAngles=[0 0 0]  RotationSequenceAnglesUnits=deg  RotationMatrix=[1 0 0; 0 1 0; 0 0 1]
  Tunnel_Thruster_Prop : Subsystem
  Tunnel_Thruster_Prop_Hub_Bearing_1 : Subsystem
  Tunnel_Thruster_Prop_Hub_Bearing_2 : Subsystem
  F : PMIOPort  Side=Left
  connections:
  T4/RConn1 -- Tunnel_Thruster_Prop/LConn1
  T3/RConn1 -- Tunnel_Thruster_Prop_Hub_Bearing_2/LConn1
  T2/RConn1 -- Tunnel_Thruster_Prop_Hub_Bearing_1/LConn1
  T1/RConn1 -- F/RConn1
  ReferenceFrame/RConn1 -- T2/LConn1 -- T4/LConn1 -- T3/LConn1 -- T1/LConn1

== system AUV_MechanicsFullHydrodynamicsVAR/AUV/Muiltibody/AUV Mechanics/BowVerThruster ==
  ReferenceFrame : sm_lib/Frames and Transforms/Reference Frame
  T1 : sm_lib/Frames and Transforms/Rigid Transform  TranslationMethod=Cartesian  TranslationStandardOffset=0  TranslationLengthUnit=m  TranslationStandardAxis=+Z  TranslationCartesianOffset=smiData.RigidTransform(4).translation  TranslationROffset=0  TranslationROffsetUnits=m  TranslationZOffset=0  TranslationZOffsetUnits=m  TranslationThetaOffset=0  TranslationThetaOffsetUnits=deg  RotationMethod=ArbitraryAxis  RotationAngleUnits=rad  RotationStandardAxis=+Z  RotationAngle=smiData.RigidTransform(4).angle  RotationArbitraryAxis=smiData.RigidTransform(4).axis  FollAlignAxisA=+X  BaseAlignAxisA=+Y  FollAlignAxisB=+Y  BaseAlignAxisB=+Z  RotationSequenceAxes=FollowerAxes  RotationSequence=XYX  RotationSequenceAngles=[0 0 0]  RotationSequenceAnglesUnits=deg  RotationMatrix=[1 0 0; 0 1 0; 0 0 1]
  T2 : sm_lib/Frames and Transforms/Rigid Transform  TranslationMethod=Cartesian  TranslationStandardOffset=0  TranslationLengthUnit=m  TranslationStandardAxis=+Z  TranslationCartesianOffset=smiData.RigidTransform(111).translation  TranslationROffset=0  TranslationROffsetUnits=m  TranslationZOffset=0  TranslationZOffsetUnits=m  TranslationThetaOffset=0  TranslationThetaOffsetUnits=deg  RotationMethod=ArbitraryAxis  RotationAngleUnits=rad  RotationStandardAxis=+Z  RotationAngle=smiData.RigidTransform(111).angle  RotationArbitraryAxis=smiData.RigidTransform(111).axis  FollAlignAxisA=+X  BaseAlignAxisA=+Y  FollAlignAxisB=+Y  BaseAlignAxisB=+Z  RotationSequenceAxes=FollowerAxes  RotationSequence=XYX  RotationSequenceAngles=[0 0 0]  RotationSequenceAnglesUnits=deg  RotationMatrix=[1 0 0; 0 1 0; 0 0 1]
  T3 : sm_lib/Frames and Transforms/Rigid Transform  TranslationMethod=Cartesian  TranslationStandardOffset=0  TranslationLengthUnit=m  TranslationStandardAxis=+Z  TranslationCartesianOffset=smiData.RigidTransform(112).translation  TranslationROffset=0  TranslationROffsetUnits=m  TranslationZOffset=0  TranslationZOffsetUnits=m  TranslationThetaOffset=0  TranslationThetaOffsetUnits=deg  RotationMethod=ArbitraryAxis  RotationAngleUnits=rad  RotationStandardAxis=+Z  RotationAngle=smiData.RigidTransform(112).angle  RotationArbitraryAxis=smiData.RigidTransform(112).axis  FollAlignAxisA=+X  BaseAlignAxisA=+Y  FollAlignAxisB=+Y  BaseAlignAxisB=+Z  RotationSequenceAxes=FollowerAxes  RotationSequence=XYX  RotationSequenceAngles=[0 0 0]  RotationSequenceAnglesUnits=deg  RotationMatrix=[1 0 0; 0 1 0; 0 0 1]
  T4 : sm_lib/Frames and Transforms/Rigid Transform  TranslationMethod=Cartesian  TranslationStandardOffset=0  TranslationLengthUnit=m  TranslationStandardAxis=+Z  TranslationCartesianOffset=smiData.RigidTransform(113).translation  TranslationROffset=0  TranslationROffsetUnits=m  TranslationZOffset=0  TranslationZOffsetUnits=m  TranslationThetaOffset=0  TranslationThetaOffsetUnits=deg  RotationMethod=ArbitraryAxis  RotationAngleUnits=rad  RotationStandardAxis=+Z  RotationAngle=smiData.RigidTransform(113).angle  RotationArbitraryAxis=smiData.RigidTransform(113).axis  FollAlignAxisA=+X  BaseAlignAxisA=+Y  FollAlignAxisB=+Y  BaseAlignAxisB=+Z  RotationSequenceAxes=FollowerAxes  RotationSequence=XYX  RotationSequenceAngles=[0 0 0]  RotationSequenceAnglesUnits=deg  RotationMatrix=[1 0 0; 0 1 0; 0 0 1]
  Tunnel_Thruster_Prop : Subsystem
  Tunnel_Thruster_Prop_Hub_Bearing_1 : Subsystem
  Tunnel_Thruster_Prop_Hub_Bearing_2 : Subsystem
  F : PMIOPort  Side=Left
  connections:
  T4/RConn1 -- Tunnel_Thruster_Prop_Hub_Bearing_2/LConn1
  T3/RConn1 -- Tunnel_Thruster_Prop/LConn1
  T2/RConn1 -- Tunnel_Thruster_Prop_Hub_Bearing_1/LConn1
  T1/RConn1 -- F/RConn1
  ReferenceFrame/RConn1 -- T2/LConn1 -- T4/LConn1 -- T3/LConn1 -- T1/LConn1

== system AUV_MechanicsFullHydrodynamicsVAR/AUV/Muiltibody/AUV Mechanics/CoMmeas ==
  " CoM Measurements" : Subsystem
      settings: PortSchema="{\"entries\":[{\"content\":{\"sides\":[{\"content\":{\"connectorIds\":[]},\"type\":\"ConnectorPlacement.EquallySpacedRectSide\",\"uuid\":\"41b17865-a6b4-4c1a-ad12-0699c57309aa\"},{\"content\":{\"connectorIds\":[\"Out1\",\"Out2\"],\"side\":\"RIGHT\"},\"type\":\"ConnectorPlacement.EquallySpacedRectSide\",\"uuid\":\"edfedad4-b08a-45ae-9215-ce29af402ac0\"},{\"content\":{\"connectorIds\":[\"LConn1\"],\"side\":\"TOP\"},\"type\":\"ConnectorPlacement.EquallySpacedRectSide\",\"uuid\":\"e431dbfc-8157-4a96-9a26-4b41afc24a27\"}]},\"type\":\"ConnectorPlacement.EquallySpacedConnector\",\"uuid\":\"fb33b9ce-c03b-4394-a7d9-78d177de3027\"}],\"packageUris\":[\"http://schema.mathworks.com/mf0/Connector/19700101\"],\"version\":\"1.0\"}"
  Derived Measurements : Subsystem
  F : PMIOPort  Side=Left
  B : PMIOPort  Port=2  Side=Right
  Out Bus Element1 : Outport  PortName=CoM  Element=Body
  Out Bus Element2 : Outport  PortName=CoM  Element=Derived
  Out Bus Element : Outport  PortName=CoM  Element=World
  wires:
  " CoM Measurements"/2(World) -> Derived Measurements/2(World), Out Bus Element/1
  " CoM Measurements"/1(Body) -> Derived Measurements/1(Body), Out Bus Element1/1
  Derived Measurements/1(Derived) -> Out Bus Element2/1
  connections:
  F/RConn1 -- " CoM Measurements"/LConn1 -- B/RConn1

== system AUV_MechanicsFullHydrodynamicsVAR/AUV/Muiltibody/AUV Mechanics/IMUmeas ==
  Measurements (wrt IMU) : sm_lib/Frames and Transforms/Transform Sensor  MeasurementFrame=NonRotatingFollower  SenseAngle=off  SenseAxis=off  SenseAngle1=off  SenseAngle2=off  SenseAngle3=off  SenseQ=off  SenseR=off  SenseOmegaX=on  SenseOmegaY=on  SenseOmegaZ=on  SenseOmega1=off  SenseOmega2=off  SenseOmega3=off  SenseQDot=off  SenseRDot=off  SenseAlphaX=off  SenseAlphaY=off  SenseAlphaZ=off  SenseAlpha1=off  SenseAlpha2=off  SenseAlpha3=off  SenseQDDot=off  SenseRDDot=off  SenseX=off  SenseY=off  SenseZ=off  SenseRad=off  SenseAzim=off  SenseDist=off  SenseInc=off  SenseXDot=off  SenseYDot=off  SenseZDot=off  SenseRadDot=off  SenseAzimDot=off  SenseDistDot=off  SenseIncDot=off  SenseXDDot=on  SenseYDDot=on  SenseZDDot=on  SenseRadDDot=off  SenseAzimDDot=off  SenseDistDDot=off  SenseIncDDot=off
  PSS1 : nesl_utility/PS-Simulink Converter  PhysicalDomain=network_engine_domain  SubClassName=ps_output  LeftPortType=input  RightPortType=output  PseudoPeriodic=off  Frequencies=[]  Unit=rad/s  AffineConversion=off
  PSS2 : nesl_utility/PS-Simulink Converter  PhysicalDomain=network_engine_domain  SubClassName=ps_output  LeftPortType=input  RightPortType=output  PseudoPeriodic=off  Frequencies=[]  Unit=rad/s  AffineConversion=off
  PSS3 : nesl_utility/PS-Simulink Converter  PhysicalDomain=network_engine_domain  SubClassName=ps_output  LeftPortType=input  RightPortType=output  PseudoPeriodic=off  Frequencies=[]  Unit=rad/s  AffineConversion=off
  PSS4 : nesl_utility/PS-Simulink Converter  PhysicalDomain=network_engine_domain  SubClassName=ps_output  LeftPortType=input  RightPortType=output  PseudoPeriodic=off  Frequencies=[]  Unit=m/s^2  AffineConversion=off
  PSS5 : nesl_utility/PS-Simulink Converter  PhysicalDomain=network_engine_domain  SubClassName=ps_output  LeftPortType=input  RightPortType=output  PseudoPeriodic=off  Frequencies=[]  Unit=m/s^2  AffineConversion=off
  PSS6 : nesl_utility/PS-Simulink Converter  PhysicalDomain=network_engine_domain  SubClassName=ps_output  LeftPortType=input  RightPortType=output  PseudoPeriodic=off  Frequencies=[]  Unit=m/s^2  AffineConversion=off
  World Frame --> e NED : sm_lib/Frames and Transforms/World Frame
  F : PMIOPort  Side=Left
  Bus Element Out : Outport  PortName=IMU  Element=p
  Out Bus Element : Outport  PortName=IMU  Element=q
  Out Bus Element1 : Outport  PortName=IMU  Element=r
  Out Bus Element2 : Outport  PortName=IMU  Element=pdot
  Out Bus Element3 : Outport  PortName=IMU  Element=qdot
  Out Bus Element4 : Outport  PortName=IMU  Element=rdot
  wires:
  PSS1/1 -> Bus Element Out/1
  PSS2/1 -> Out Bus Element/1
  PSS3/1 -> Out Bus Element1/1
  PSS4/1 -> Out Bus Element2/1
  PSS5/1 -> Out Bus Element3/1
  PSS6/1 -> Out Bus Element4/1
  connections:
  World Frame --> e NED/RConn1 -- Measurements (wrt IMU)/LConn1
  Measurements (wrt IMU)/RConn1 -- F/RConn1
  PSS1/LConn1 -- Measurements (wrt IMU)/RConn2
  PSS2/LConn1 -- Measurements (wrt IMU)/RConn3
  Measurements (wrt IMU)/RConn4 -- PSS3/LConn1
  Measurements (wrt IMU)/RConn5 -- PSS4/LConn1
  Measurements (wrt IMU)/RConn6 -- PSS5/LConn1
  Measurements (wrt IMU)/RConn7 -- PSS6/LConn1

== system AUV_MechanicsFullHydrodynamicsVAR/AUV/Muiltibody/AUV Mechanics/PortProp ==
  Main_Prop : Subsystem
  Main_Prop_Bearing : Subsystem
  Main_Prop_Driven_Hub : Subsystem
  Main_Prop_Hub : Subsystem
  Main_Prop_Hub_Bearing : Subsystem
  ReferenceFrame : sm_lib/Frames and Transforms/Reference Frame
  T1 : sm_lib/Frames and Transforms/Rigid Transform  TranslationMethod=Cartesian  TranslationStandardOffset=0  TranslationLengthUnit=m  TranslationStandardAxis=+Z  TranslationCartesianOffset=smiData.RigidTransform(8).translation  TranslationROffset=0  TranslationROffsetUnits=m  TranslationZOffset=0  TranslationZOffsetUnits=m  TranslationThetaOffset=0  TranslationThetaOffsetUnits=deg  RotationMethod=ArbitraryAxis  RotationAngleUnits=rad  RotationStandardAxis=+Z  RotationAngle=smiData.RigidTransform(8).angle  RotationArbitraryAxis=smiData.RigidTransform(8).axis  FollAlignAxisA=+X  BaseAlignAxisA=+Y  FollAlignAxisB=+Y  BaseAlignAxisB=+Z  RotationSequenceAxes=FollowerAxes  RotationSequence=XYX  RotationSequenceAngles=[0 0 0]  RotationSequenceAnglesUnits=deg  RotationMatrix=[1 0 0; 0 1 0; 0 0 1]
  T2 : sm_lib/Frames and Transforms/Rigid Transform  TranslationMethod=Cartesian  TranslationStandardOffset=0  TranslationLengthUnit=m  TranslationStandardAxis=+Z  TranslationCartesianOffset=smiData.RigidTransform(103).translation  TranslationROffset=0  TranslationROffsetUnits=m  TranslationZOffset=0  TranslationZOffsetUnits=m  TranslationThetaOffset=0  TranslationThetaOffsetUnits=deg  RotationMethod=ArbitraryAxis  RotationAngleUnits=rad  RotationStandardAxis=+Z  RotationAngle=smiData.RigidTransform(103).angle  RotationArbitraryAxis=smiData.RigidTransform(103).axis  FollAlignAxisA=+X  BaseAlignAxisA=+Y  FollAlignAxisB=+Y  BaseAlignAxisB=+Z  RotationSequenceAxes=FollowerAxes  RotationSequence=XYX  RotationSequenceAngles=[0 0 0]  RotationSequenceAnglesUnits=deg  RotationMatrix=[1 0 0; 0 1 0; 0 0 1]
  T3 : sm_lib/Frames and Transforms/Rigid Transform  TranslationMethod=Cartesian  TranslationStandardOffset=0  TranslationLengthUnit=m  TranslationStandardAxis=+Z  TranslationCartesianOffset=smiData.RigidTransform(104).translation  TranslationROffset=0  TranslationROffsetUnits=m  TranslationZOffset=0  TranslationZOffsetUnits=m  TranslationThetaOffset=0  TranslationThetaOffsetUnits=deg  RotationMethod=ArbitraryAxis  RotationAngleUnits=rad  RotationStandardAxis=+Z  RotationAngle=smiData.RigidTransform(104).angle  RotationArbitraryAxis=smiData.RigidTransform(104).axis  FollAlignAxisA=+X  BaseAlignAxisA=+Y  FollAlignAxisB=+Y  BaseAlignAxisB=+Z  RotationSequenceAxes=FollowerAxes  RotationSequence=XYX  RotationSequenceAngles=[0 0 0]  RotationSequenceAnglesUnits=deg  RotationMatrix=[1 0 0; 0 1 0; 0 0 1]
  T4 : sm_lib/Frames and Transforms/Rigid Transform  TranslationMethod=Cartesian  TranslationStandardOffset=0  TranslationLengthUnit=m  TranslationStandardAxis=+Z  TranslationCartesianOffset=smiData.RigidTransform(105).translation  TranslationROffset=0  TranslationROffsetUnits=m  TranslationZOffset=0  TranslationZOffsetUnits=m  TranslationThetaOffset=0  TranslationThetaOffsetUnits=deg  RotationMethod=ArbitraryAxis  RotationAngleUnits=rad  RotationStandardAxis=+Z  RotationAngle=smiData.RigidTransform(105).angle  RotationArbitraryAxis=smiData.RigidTransform(105).axis  FollAlignAxisA=+X  BaseAlignAxisA=+Y  FollAlignAxisB=+Y  BaseAlignAxisB=+Z  RotationSequenceAxes=FollowerAxes  RotationSequence=XYX  RotationSequenceAngles=[0 0 0]  RotationSequenceAnglesUnits=deg  RotationMatrix=[1 0 0; 0 1 0; 0 0 1]
  T5 : sm_lib/Frames and Transforms/Rigid Transform  TranslationMethod=Cartesian  TranslationStandardOffset=0  TranslationLengthUnit=m  TranslationStandardAxis=+Z  TranslationCartesianOffset=smiData.RigidTransform(106).translation  TranslationROffset=0  TranslationROffsetUnits=m  TranslationZOffset=0  TranslationZOffsetUnits=m  TranslationThetaOffset=0  TranslationThetaOffsetUnits=deg  RotationMethod=ArbitraryAxis  RotationAngleUnits=rad  RotationStandardAxis=+Z  RotationAngle=smiData.RigidTransform(106).angle  RotationArbitraryAxis=smiData.RigidTransform(106).axis  FollAlignAxisA=+X  BaseAlignAxisA=+Y  FollAlignAxisB=+Y  BaseAlignAxisB=+Z  RotationSequenceAxes=FollowerAxes  RotationSequence=XYX  RotationSequenceAngles=[0 0 0]  RotationSequenceAnglesUnits=deg  RotationMatrix=[1 0 0; 0 1 0; 0 0 1]
  T6 : sm_lib/Frames and Transforms/Rigid Transform  TranslationMethod=Cartesian  TranslationStandardOffset=0  TranslationLengthUnit=m  TranslationStandardAxis=+Z  TranslationCartesianOffset=smiData.RigidTransform(107).translation  TranslationROffset=0  TranslationROffsetUnits=m  TranslationZOffset=0  TranslationZOffsetUnits=m  TranslationThetaOffset=0  TranslationThetaOffsetUnits=deg  RotationMethod=ArbitraryAxis  RotationAngleUnits=rad  RotationStandardAxis=+Z  RotationAngle=smiData.RigidTransform(107).angle  RotationArbitraryAxis=smiData.RigidTransform(107).axis  FollAlignAxisA=+X  BaseAlignAxisA=+Y  FollAlignAxisB=+Y  BaseAlignAxisB=+Z  RotationSequenceAxes=FollowerAxes  RotationSequence=XYX  RotationSequenceAngles=[0 0 0]  RotationSequenceAnglesUnits=deg  RotationMatrix=[1 0 0; 0 1 0; 0 0 1]
  T7 : sm_lib/Frames and Transforms/Rigid Transform  TranslationMethod=None  TranslationStandardOffset=0  TranslationLengthUnit=m  TranslationStandardAxis=+Z  TranslationCartesianOffset=[0 0 0]  TranslationROffset=0  TranslationROffsetUnits=m  TranslationZOffset=0  TranslationZOffsetUnits=m  TranslationThetaOffset=0  TranslationThetaOffsetUnits=deg  RotationMethod=RotationSequence  RotationAngleUnits=deg  RotationStandardAxis=+X  RotationAngle=180.0  RotationArbitraryAxis=[0 0 1]  FollAlignAxisA=+X  BaseAlignAxisA=+Y  FollAlignAxisB=+Y  BaseAlignAxisB=+Z  RotationSequenceAxes=BaseAxes  RotationSequence=XZX  RotationSequenceAngles=[180 -90 0]  RotationSequenceAnglesUnits=deg  RotationMatrix=[1 0 0; 0 1 0; 0 0 1]
  F : PMIOPort  Side=Left
  connections:
  Main_Prop_Driven_Hub/LConn1 -- T6/RConn1
  Main_Prop_Bearing/LConn1 -- T5/RConn1
  Main_Prop_Hub/LConn1 -- T4/RConn1
  Main_Prop_Hub_Bearing/LConn1 -- T3/RConn1
  Main_Prop/LConn1 -- T2/RConn1
  F/RConn1 -- T7/RConn1
  ReferenceFrame/RConn1 -- T2/LConn1 -- T4/LConn1 -- T6/LConn1 -- T5/LConn1 -- T3/LConn1 -- T1/LConn1
  T1/RConn1 -- T7/LConn1
